simulink model "Decentralized_Control_G18_2017"  (R2017a)
settings: Solver=VariableStepAuto  StartTime=0.0  StopTime=35  RelTol=1e-3
values from neighbouring files (symbols this model uses):
  DH = Robot_G18()    [Kinematics_G18.m]
undefined symbols (not defined in the file or in its folder): DK_dH, DK_pH
libraries: vrlib x7, simulink_extras x3, dspinverses x2, aerolibanimutils x1, RobotG18_Blocos x1, simulink x1
settings Model: Creator=Ricardo Henriques  LastModifiedBy=Catarina
settings OptimizationCC: LifeSpan=inf

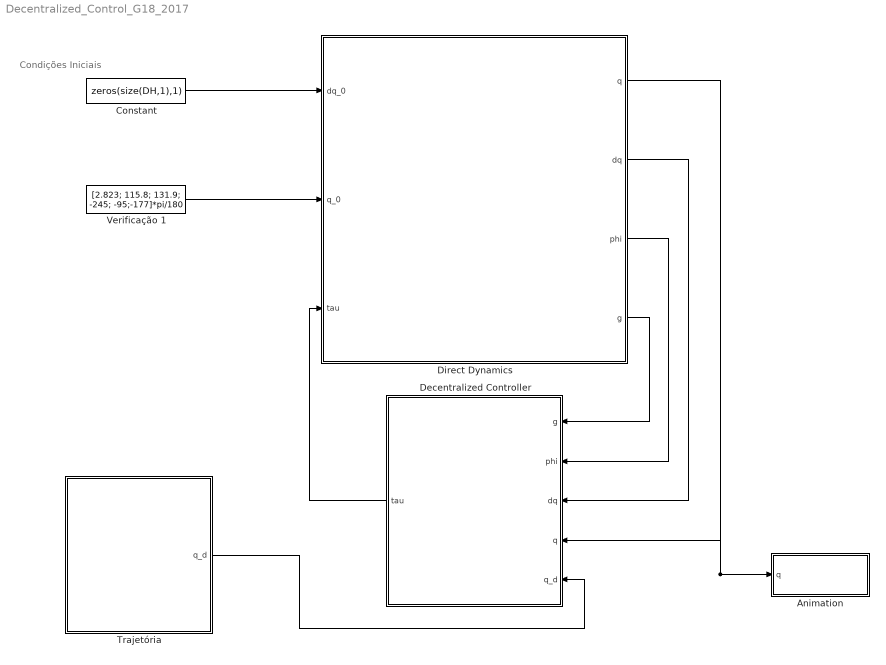
== system Decentralized_Control_G18_2017 ==
  note: Condições Iniciais
  "Animation " : Subsystem
  Constant : Constant  Value=zeros(size(DH,1),1)  VectorParams1D=off
  Decentralized Controller : Subsystem
  Direct Dynamics : Subsystem
  Trajetória : Subsystem
  Verificação 1 : Constant  Value=[2.823; 115.8; 131.9; -245; -95;-177]*pi/180  VectorParams1D=off
  wires:
  Constant/1 -> Direct Dynamics/1(dq_0)
  Direct Dynamics/4(g) -> Decentralized Controller/1(g)
  Direct Dynamics/3(phi) -> Decentralized Controller/2("phi ")
  Decentralized Controller/1(tau) -> Direct Dynamics/3(tau)
  Trajetória/1(q_d) -> Decentralized Controller/5(q_d)
  Verificação 1/1 -> Direct Dynamics/2(q_0)
  Direct Dynamics/2(dq) -> Decentralized Controller/3(dq)
  Direct Dynamics/1(q) -> Decentralized Controller/4(q), "Animation "/1("q ")

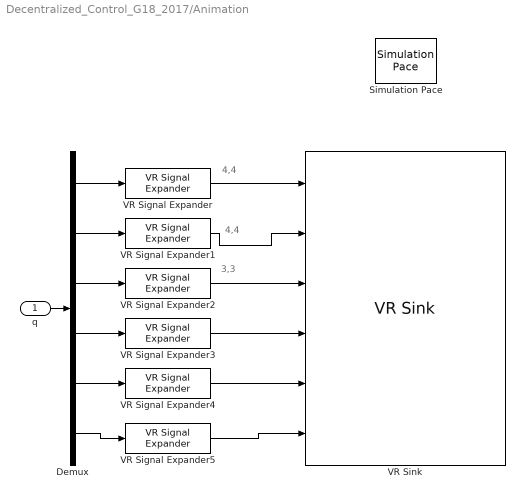
== system Decentralized_Control_G18_2017/Animation  ==
  note: 4,4
  note: 3,3
  note: 4,4
  "q " : Inport
  Demux : Demux  Outputs=6
  Simulation Pace : aerolibanimutils/Simulation Pace  SimulationPace=1  SleepMode=Auto  OutputPaceError=off  SampleTime=1/30
  VR Signal Expander{,1..5} (6 alike) : vrlib/VR Signal Expander  outwidth=4  outidx=4
  VR Sink : vrlib/VR Sink  InstantiateOnLoad=on  SampleTime=1/30  ViewEnable=on  RemoteChange=off  RemoteView=off  FieldsWritten=Jt1_DH_dv.rotation.4.1.1.double#Jt2_DH_dv.rotation.4.1.1.double#Jt3_DH_dv.rotation.4.1.1.double#Jt4_DH_dv.rotation.4.1.1.double#Jt5_DH_dv.rotation.4.1.1.double#Jt6_DH_dv.rotation.4.1.1.double  WorldFileName=RobotG18_Opt_NoAxes.wrl  WorldDescription=D-H Reference Frames for Virtual Reality Robot  AutoView=off  VideoDimensions=[]  AllowVariableSize=off
  wires:
  "q "/1 -> Demux/1
  Demux/1 -> VR Signal Expander/1
  Demux/2 -> VR Signal Expander1/1
  Demux/3 -> VR Signal Expander2/1
  Demux/4 -> VR Signal Expander3/1
  Demux/5 -> VR Signal Expander4/1
  Demux/6 -> VR Signal Expander5/1
  VR Signal Expander/1 -> VR Sink/1
  VR Signal Expander1/1 -> VR Sink/2
  VR Signal Expander5/1 -> VR Sink/6
  VR Signal Expander2/1 -> VR Sink/3
  VR Signal Expander3/1 -> VR Sink/4
  VR Signal Expander4/1 -> VR Sink/5

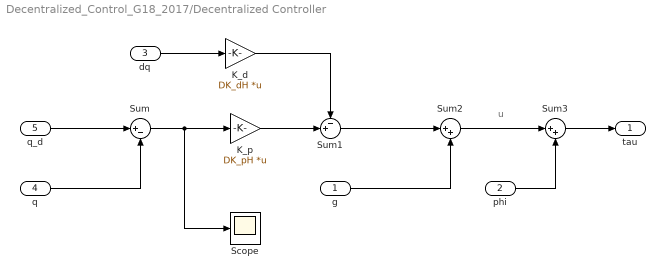
== system Decentralized_Control_G18_2017/Decentralized Controller ==
  note: u
  g : Inport
  "phi " : Inport  Port=2
  dq : Inport  Port=3
  q : Inport  Port=4
  q_d : Inport  Port=5
  K_d : Gain  Gain=DK_dH  Multiplication=Matrix(K*u) (u vector)
  K_p : Gain  Gain=DK_pH  Multiplication=Matrix(K*u) (u vector)
  Scope : Scope
  Sum : Sum  Inputs=|+-
  Sum1 : Sum  Inputs=-+|
  Sum2 : Sum  Inputs=|++
  Sum3 : Sum  Inputs=|++
  tau : Outport
  wires:
  q_d/1 -> Sum/1
  Sum1/1 -> Sum2/1
  g/1 -> Sum2/2
  Sum3/1 -> tau/1
  "phi "/1 -> Sum3/2
  Sum2/1 -> Sum3/1
  q/1 -> Sum/2
  dq/1 -> K_d/1
  K_d/1 -> Sum1/1
  K_p/1 -> Sum1/2
  Sum/1 -> Scope/1, K_p/1

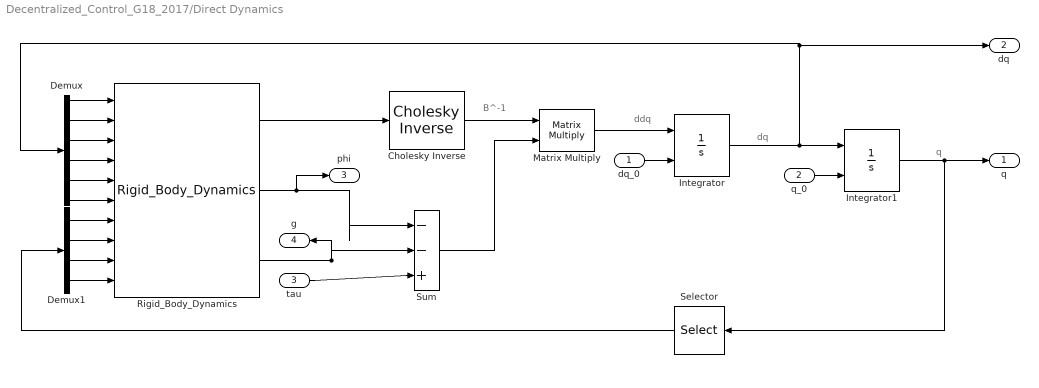
== system Decentralized_Control_G18_2017/Direct Dynamics ==
  note: q
  note: dq
  note: ddq
  note: B^-1
  dq_0 : Inport
  q_0 : Inport  Port=2
  tau : Inport  Port=3
  Cholesky Inverse : dspinverses/Cholesky Inverse  errmode=Warning
      settings: SourceProductBaseCode=DS
  Demux : Demux  Outputs=6
  Demux1 : Demux
  Integrator : Integrator  InitialConditionSource=external
  Integrator1 : Integrator  InitialConditionSource=external
  Matrix Multiply : Product  Multiplication=Matrix(*)
  Rigid_Body_Dynamics : RobotG18_Blocos/Rigid_Body_Dynamics  SystemSampleTime=-1  Latency=0  AutoFrameSizeCalculation=off
  Selector : Selector  InputPortWidth=6  IndexOptions=Index vector (dialog)  Indices=[2 3 4 5]  OutputSizes=1
  Sum : Sum  Inputs=|--+
  q : Outport
  dq : Outport  Port=2
  phi : Outport  Port=3
  g : Outport  Port=4
  wires:
  dq_0/1 -> Integrator/2
  Integrator1/1 -> q/1, Selector/1
  Integrator/1 -> Demux/1, dq/1, Integrator1/1
  q_0/1 -> Integrator1/2
  Matrix Multiply/1 -> Integrator/1
  Cholesky Inverse/1 -> Matrix Multiply/1
  Sum/1 -> Matrix Multiply/2
  Rigid_Body_Dynamics/1 -> Cholesky Inverse/1
  tau/1 -> Sum/3
  Rigid_Body_Dynamics/3 -> g/1, Sum/2
  Rigid_Body_Dynamics/2 -> phi/1, Sum/1
  Demux/1 -> Rigid_Body_Dynamics/1
  Demux/2 -> Rigid_Body_Dynamics/2
  Demux/3 -> Rigid_Body_Dynamics/3
  Demux/4 -> Rigid_Body_Dynamics/4
  Demux/5 -> Rigid_Body_Dynamics/5
  Demux/6 -> Rigid_Body_Dynamics/6
  Demux1/1 -> Rigid_Body_Dynamics/7
  Demux1/2 -> Rigid_Body_Dynamics/8
  Demux1/3 -> Rigid_Body_Dynamics/9
  Demux1/4 -> Rigid_Body_Dynamics/10
  Selector/1 -> Demux1/1

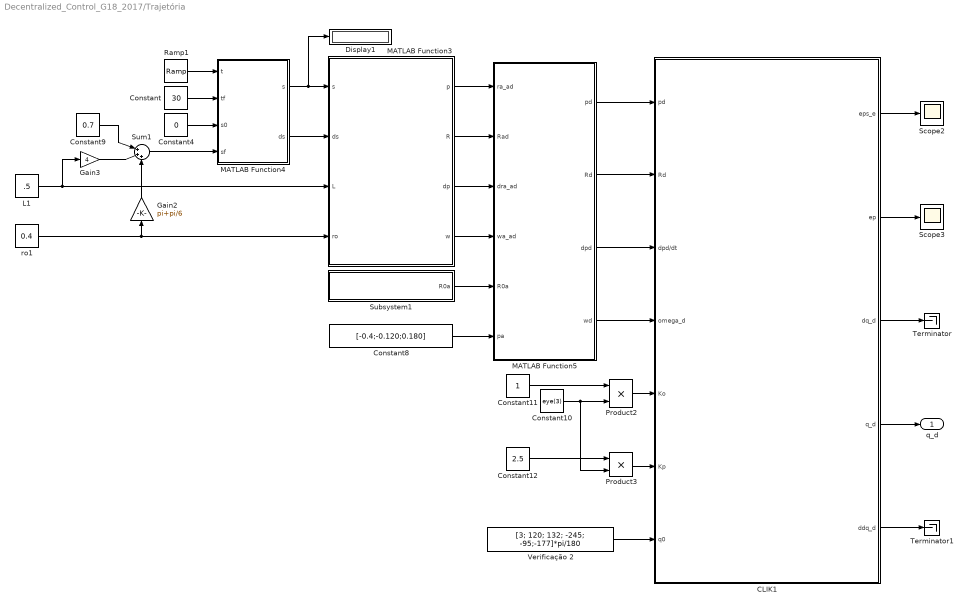
== system Decentralized_Control_G18_2017/Trajetória ==
  CLIK1 : Subsystem
  Constant : Constant  Value=30
  Constant10 : Constant  Value=eye(3)
  Constant11 : Constant
  Constant12 : Constant  Value=2.5
  Constant4 : Constant  Value=0
  Constant8 : Constant  Value=[-0.4;-0.120;0.180]  VectorParams1D=off
  Constant9 : Constant  Value=0.7
  Display1 : Display
  Gain2 : Gain  Gain=pi+pi/6
  Gain3 : Gain  Gain=4
  L1 : Constant  Value=.5
  MATLAB Function3 : MATLAB Function  TreatAsAtomicUnit=on
  MATLAB Function4 : MATLAB Function  TreatAsAtomicUnit=on
  MATLAB Function5 : MATLAB Function  TreatAsAtomicUnit=on
  Product2 : Product
  Product3 : Product
  Ramp1 : simulink/Sources/Ramp  slope=1  start=0  X0=0
  Scope2 : Scope
  Scope3 : Scope
  Subsystem1 : Subsystem
  Sum1 : Sum  Inputs=|+++
  Terminator : Terminator
  Terminator1 : Terminator
  Verificação 2 : Constant  Value=[3; 120; 132; -245; -95;-177]*pi/180  VectorParams1D=off  SampleTime=inf
  ro1 : Constant  Value=0.4
  q_d : Outport
  wires:
  MATLAB Function5/4(wd) -> CLIK1/4(omega_d)
  Constant8/1 -> MATLAB Function5/6(pa)
  Constant10/1 -> Product3/2, Product2/2
  CLIK1/4(q_d) -> q_d/1
  CLIK1/2(ep) -> Scope3/1
  MATLAB Function5/3(dpd) -> CLIK1/3(dpd/dt)
  CLIK1/1(eps_e) -> Scope2/1
  Product2/1 -> CLIK1/5(Ko)
  MATLAB Function3/3(dp) -> MATLAB Function5/3(dra_ad)
  ro1/1 -> MATLAB Function3/4(ro), Gain2/1
  MATLAB Function4/2(ds) -> MATLAB Function3/2(ds)
  Constant9/1 -> Sum1/1
  Constant4/1 -> MATLAB Function4/3(s0)
  Sum1/1 -> MATLAB Function4/4(sf)
  MATLAB Function5/1(pd) -> CLIK1/1(pd)
  L1/1 -> MATLAB Function3/3(L), Gain3/1
  Constant/1 -> MATLAB Function4/2(tf)
  MATLAB Function4/1(s) -> Display1/1, MATLAB Function3/1(s)
  Gain2/1 -> Sum1/3
  MATLAB Function3/4(w) -> MATLAB Function5/4(wa_ad)
  Ramp1/1 -> MATLAB Function4/1(t)
  MATLAB Function5/2(Rd) -> CLIK1/2(Rd)
  Gain3/1 -> Sum1/2
  Constant12/1 -> Product3/1
  MATLAB Function3/1(p) -> MATLAB Function5/1(ra_ad)
  MATLAB Function3/2(R) -> MATLAB Function5/2(Rad)
  Product3/1 -> CLIK1/6(Kp)
  Constant11/1 -> Product2/1
  Subsystem1/1(R0a) -> MATLAB Function5/5(R0a)
  Verificação 2/1 -> CLIK1/7(q0)
  CLIK1/3(dq_d) -> Terminator/1
  CLIK1/5(ddq_d) -> Terminator1/1

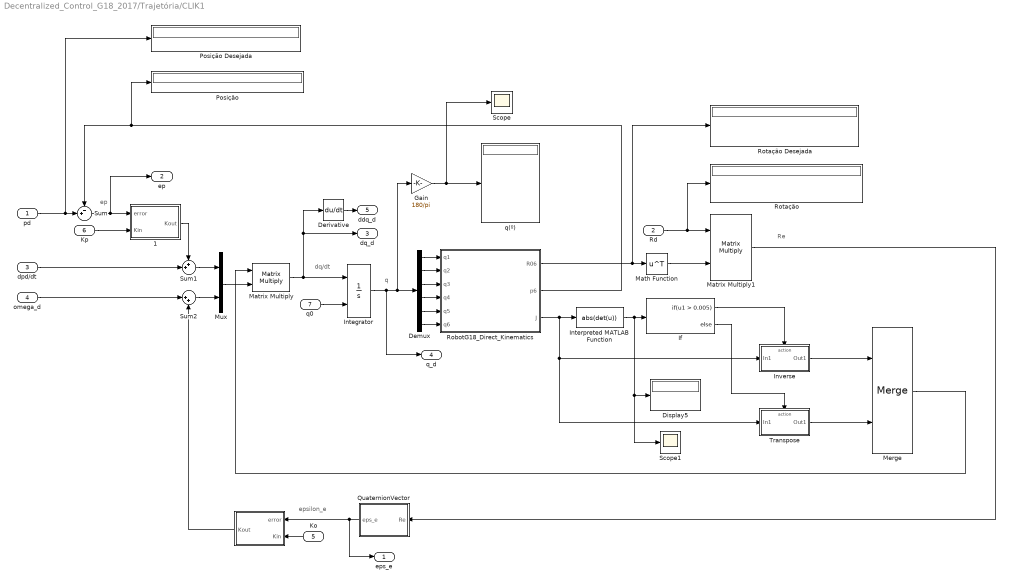
== system Decentralized_Control_G18_2017/Trajetória/CLIK1 ==
  note: epsilon_e
  note: Re
  note: ep
  note: dq/dt
  note: q
  pd : Inport
  Rd : Inport  Port=2
  dpd/dt : Inport  Port=3
  omega_d : Inport  Port=4
  Ko : Inport  Port=5
  Kp : Inport  Port=6
  q0 : Inport  Port=7
  " " : MATLAB Function  TreatAsAtomicUnit=on
  " 1" : MATLAB Function  TreatAsAtomicUnit=on
  Demux : Demux  Outputs=6
  Derivative : Derivative
  Display5 : Display
  Gain : Gain  Gain=180/pi
  If : If  IfExpression=u1 > 0.005  ZeroCross=off
  Integrator : Integrator  InitialConditionSource=external
  Interpreted MATLAB Function : MATLABFcn  MATLABFcn=abs(det(u))
  Inverse : Subsystem  TreatAsAtomicUnit=on
  Math Function : Math  Operator=transpose  SaturateOnIntegerOverflow=on
  Matrix Multiply : Product  Multiplication=Matrix(*)
  Matrix Multiply1 : Product  Multiplication=Matrix(*)
  Merge : Merge
  Mux : Mux  Inputs=2
  Posição : Display
      settings: Decimation=3
  Posição Desejada : Display
      settings: Decimation=3
  QuaternionVector : MATLAB Function  TreatAsAtomicUnit=on
  RobotG18_Direct_Kinematics : MATLAB Function  TreatAsAtomicUnit=on
  Rotação : Display
      settings: Decimation=3
  Rotação Desejada : Display
      settings: Decimation=3
  Scope : Scope
  Scope1 : Scope
  Sum : Sum  Inputs=-+|
  Sum1 : Sum  Inputs=++|
  Sum2 : Sum  Inputs=|++
  Transpose : Subsystem  TreatAsAtomicUnit=on
  q(º) : Display
  eps_e : Outport
  ep : Outport  Port=2
  dq_d : Outport  Port=3
  q_d : Outport  Port=4
  ddq_d : Outport  Port=5
  wires:
  Integrator/1 -> q_d/1, Gain/1, Demux/1
  Demux/3 -> RobotG18_Direct_Kinematics/3(q3)
  Demux/4 -> RobotG18_Direct_Kinematics/4(q4)
  Demux/1 -> RobotG18_Direct_Kinematics/1(q1)
  Demux/2 -> RobotG18_Direct_Kinematics/2(q2)
  Demux/5 -> RobotG18_Direct_Kinematics/5(q5)
  Demux/6 -> RobotG18_Direct_Kinematics/6(q6)
  QuaternionVector/1(eps_e) -> " "/1(error), eps_e/1
  Matrix Multiply/1 -> Derivative/1, dq_d/1, Integrator/1
  Math Function/1 -> Matrix Multiply1/2
  " "/1(Kout) -> Sum2/2
  omega_d/1 -> Sum2/1
  Sum2/1 -> Mux/2
  Sum1/1 -> Mux/1
  Mux/1 -> Matrix Multiply/2
  Rd/1 -> Rotação/1, Matrix Multiply1/1
  Matrix Multiply1/1 -> QuaternionVector/1(Re)
  pd/1 -> Posição Desejada/1, Sum/2
  RobotG18_Direct_Kinematics/2(p6) -> Posição/1, Sum/1
  Sum/1 -> " 1"/1(error), ep/1
  dpd/dt/1 -> Sum1/2
  RobotG18_Direct_Kinematics/1(R06) -> Math Function/1, Rotação Desejada/1
  RobotG18_Direct_Kinematics/3(J) -> Interpreted MATLAB Function/1, Inverse/1(In1), Transpose/1(In1)
  If/1 -> Inverse/Action
  If/2 -> Transpose/Action
  Transpose/1(Out1) -> Merge/2
  Inverse/1(Out1) -> Merge/1
  Merge/1 -> Matrix Multiply/1
  Gain/1 -> Scope/1, q(º)/1
  q0/1 -> Integrator/2
  Ko/1 -> " "/2(Kin)
  " 1"/1(Kout) -> Sum1/1
  Kp/1 -> " 1"/2(Kin)
  Interpreted MATLAB Function/1 -> Scope1/1, Display5/1, If/1
  Derivative/1 -> ddq_d/1

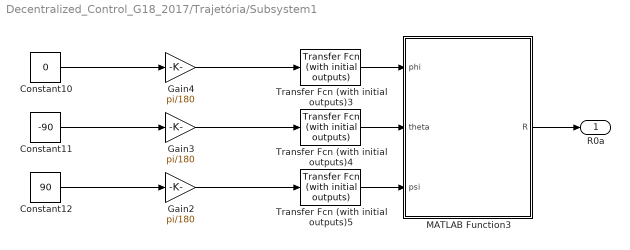
== system Decentralized_Control_G18_2017/Trajetória/Subsystem1 ==
  Constant10 : Constant  Value=0
  Constant11 : Constant  Value=-90
  Constant12 : Constant  Value=90
  Gain2 : Gain  Gain=pi/180
  Gain3 : Gain  Gain=pi/180
  Gain4 : Gain  Gain=pi/180
  MATLAB Function3 : MATLAB Function  TreatAsAtomicUnit=on
  Transfer Fcn (with initial outputs)3 : simulink_extras/Additional Linear/Transfer Fcn (with initial outputs)  N=[2]  D="[1  2]"  Y0=0  U0=0
  Transfer Fcn (with initial outputs)4 : simulink_extras/Additional Linear/Transfer Fcn (with initial outputs)  N=[2]  D="[1  2]"  Y0=-90  U0=0
  Transfer Fcn (with initial outputs)5 : simulink_extras/Additional Linear/Transfer Fcn (with initial outputs)  N=[2]  D="[1  2]"  Y0=90  U0=0
  R0a : Outport
  wires:
  Gain3/1 -> Transfer Fcn (with initial outputs)4/1
  Gain2/1 -> Transfer Fcn (with initial outputs)5/1
  Gain4/1 -> Transfer Fcn (with initial outputs)3/1
  Constant10/1 -> Gain4/1
  Transfer Fcn (with initial outputs)4/1 -> MATLAB Function3/2(theta)
  Transfer Fcn (with initial outputs)5/1 -> MATLAB Function3/3(psi)
  Transfer Fcn (with initial outputs)3/1 -> MATLAB Function3/1(phi)
  Constant11/1 -> Gain3/1
  Constant12/1 -> Gain2/1
  MATLAB Function3/1(R) -> R0a/1

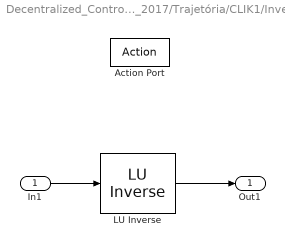
== system Decentralized_Control_G18_2017/Trajetória/CLIK1/Inverse ==
  In1 : Inport
  Action Port : ActionPort
  " LU Inverse" : dspinverses/ LU Inverse
  Out1 : Outport
  wires:
  In1/1 -> " LU Inverse"/1
  " LU Inverse"/1 -> Out1/1

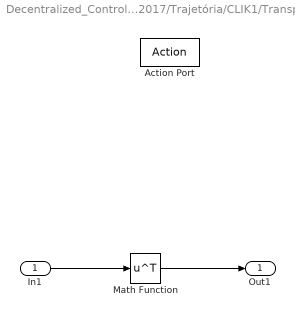
== system Decentralized_Control_G18_2017/Trajetória/CLIK1/Transpose ==
  In1 : Inport
  Action Port : ActionPort
  Math Function : Math  Operator=transpose  SaturateOnIntegerOverflow=on
  Out1 : Outport
  wires:
  In1/1 -> Math Function/1
  Math Function/1 -> Out1/1

== matlab function Decentralized_Control_G18_2017/Trajetória/CLIK1/  ==
  data: error input; Kin input; Kout output
function Kout = Gains(error, Kin)

Kout = Kin*error;

== matlab function Decentralized_Control_G18_2017/Trajetória/CLIK1/ 1 ==
  data: error input; Kin input; Kout output
function Kout = Gains(error, Kin)

Kout = Kin*error;

== matlab function Decentralized_Control_G18_2017/Trajetória/CLIK1/QuaternionVector ==
  data: Re input; eps_e output
function eps_e  = QuaternionVector(Re)

eps_e = 0.5 * [sign(Re(3,2)-Re(2,3)) * sqrt(abs(Re(1,1)-Re(2,2)-Re(3,3)+1));
               sign(Re(1,3)-Re(3,1)) * sqrt(abs(Re(2,2)-Re(1,1)-Re(3,3)+1));
               sign(Re(2,1)-Re(1,2)) * sqrt(abs(Re(3,3)-Re(1,1)-Re(2,2)+1))];
           
end

== matlab function Decentralized_Control_G18_2017/Trajetória/CLIK1/RobotG18_Direct_Kinematics ==
  data: q1 input; R06 output; q2 input; q3 input; q4 input; q5 input; q6 input; p6 output; J output
function [R06,p6,J] = RobotG18_Direct_Kinematics(q1,q2,q3,q4,q5,q6)
%#codegen

%    This function was generated by the Symbolic Math Toolbox version 7.0.
%    15-Apr-2021 18:49:51

t2 = q2+q3+q4;
t3 = cos(q1);
t4 = sin(q6);
t5 = sin(q1);
t6 = sin(q5);
t7 = t5.*t6;
t8 = cos(t2);
t9 = cos(q5);
t10 = t7-t3.*t8.*t9;
t11 = sin(t2);
t12 = cos(q6);
t13 = t3.*t6;
t14 = t5.*t8.*t9;
t15 = t13+t14;
t16 = q2+q3;
t17 = cos(q2);
t18 = sin(q2);
t19 = sin(q3);
t20 = cos(t16);
t21 = sin(q4);
t22 = sin(t16);
t23 = cos(q4);
t24 = cos(q3);
t25 = t5.*t17.*(1.7e1./4.0e1);
t26 = t5.*t6.*t8.*(4.1e1./5.0e2);
t27 = t5.*t17.*t24.*(4.9e1./1.25e2);
t28 = t22.*(4.9e1./1.25e2);
t29 = t18.*(1.7e1./4.0e1);
t30 = t20.*t21.*(4.1e1./5.0e2);
t31 = t22.*t23.*(4.1e1./5.0e2);
t32 = t30+t31;
t33 = t6.*t32;
t34 = t20.*t23.*(1.9e1./2.0e2);
t35 = t8.*(1.9e1./2.0e2);
t36 = t6.*t11.*(4.1e1./5.0e2);
t37 = t5.*(1.09e2./1.0e3);
t38 = t3.*t17.*(1.7e1./4.0e1);
t39 = t5.*t9.*(4.1e1./5.0e2);
t40 = t3.*t6.*t8.*(4.1e1./5.0e2);
t41 = t3.*t17.*t24.*(4.9e1./1.25e2);
t42 = t37+t38+t39+t40+t41-t3.*t18.*t19.*(4.9e1./1.25e2)-t3.*t20.*t21.*(1.9e1./2.0e2)-t3.*t22.*t23.*(1.9e1./2.0e2);
t43 = t28+t29+t33+t34-t21.*t22.*(1.9e1./2.0e2);
t44 = t28+t35+t36;
t45 = t35+t36;
t46 = q2+q3+q4+q5;
t47 = sin(t46);
t48 = t47.*(4.1e1./1.0e3);
t49 = t20.*(4.9e1./1.25e2);
t50 = q2+q3+q4-q5;
t51 = sin(t50);
t52 = t5.*t9;
t53 = t3.*t6.*t8;
t54 = t52+t53;
t55 = t5.*t6.*t8;
t56 = t55-t3.*t9;
t57 = t6.*t11;
R06 = reshape([-t10.*t12-t3.*t4.*t11,t12.*t15-t4.*t5.*t11,t4.*t8+t9.*t11.*t12,t4.*t10-t3.*t11.*t12,-t4.*t15-t5.*t11.*t12,t8.*t12-t4.*t9.*t11,t54,t56,t57],[3,3]);
if nargout > 1
    p6 = [t42;t3.*(-1.09e2./1.0e3)+t25+t26+t27-t3.*t9.*(4.1e1./5.0e2)-t5.*t18.*t19.*(4.9e1./1.25e2)-t5.*t20.*t21.*(1.9e1./2.0e2)-t5.*t22.*t23.*(1.9e1./2.0e2);t28+t29+t33+t34-t21.*t22.*(1.9e1./2.0e2)+8.9e1./1.0e3];
end
if nargout > 2
    J = reshape([t3.*(1.09e2./1.0e3)-t25-t26-t27+t3.*t9.*(4.1e1./5.0e2)+t5.*t18.*t19.*(4.9e1./1.25e2)+t5.*t20.*t21.*(1.9e1./2.0e2)+t5.*t22.*t23.*(1.9e1./2.0e2),t42,0.0,0.0,0.0,1.0,-t3.*t43,-t5.*t43,t11.*(-1.9e1./2.0e2)+t17.*(1.7e1./4.0e1)+t48+t49-t51.*(4.1e1./1.0e3),t5,-t3,0.0,-t3.*t44,-t5.*t44,t11.*(-1.9e1./2.0e2)+t48+t49-t51.*(4.1e1./1.0e3),t5,-t3,0.0,-t3.*t45,-t5.*t45,t11.*(-1.9e1./2.0e2)+t48-t51.*(4.1e1./1.0e3),t5,-t3,0.0,t5.*t6.*(-4.1e1./5.0e2)-t3.*t9.*t17.*t19.*t21.*(4.1e1./5.0e2)-t3.*t9.*t18.*t19.*t23.*(4.1e1./5.0e2)-t3.*t9.*t18.*t21.*t24.*(4.1e1./5.0e2)+t3.*t9.*t17.*t23.*t24.*(4.1e1./5.0e2),t3.*t6.*(4.1e1./5.0e2)-t5.*t9.*t17.*t19.*t21.*(4.1e1./5.0e2)-t5.*t9.*t18.*t19.*t23.*(4.1e1./5.0e2)-t5.*t9.*t18.*t21.*t24.*(4.1e1./5.0e2)+t5.*t9.*t17.*t23.*t24.*(4.1e1./5.0e2),t48+t51.*(4.1e1./1.0e3),-t3.*t11,-t5.*t11,t8,0.0,0.0,0.0,t54,t56,t57],[6,6]);
end

== matlab function Decentralized_Control_G18_2017/Trajetória/MATLAB Function3 ==
  data: p output; R output; s input; ds input; L input; ro input; dp output; w output
function [p,R,dp,w] = trajectory(s,ds,L,ro)

p=zeros(3,1);
R=eye(3);
dp=zeros(3,1);
w=zeros(3,1);

if 0 <= s && s<= L
%% Path 1 ------- Subida ---------
    p=[0;-s;0];
    R=[1 0 0; 0 1 0; 0 0 1];
    
    dp=[0;ds;0];
    w=zeros(3,1);
    
elseif L < s && s <= L+((pi/2)*ro)
%% Path 2  ------- Roda ---------
    p=[ro*sin((s-L)/ro);
        -L;
        -ro+ro*cos((s-L)/ro)];
    
    R=[ cos((s-L)/ro)   0   sin((s-L)/ro);
        0          1          0
        -sin((s-L)/ro)   0    cos((s-L)/ro)];
    
    dp = ds*[cos((s-L)/ro);0;-sin((s-L)/ro)];
    
    dR = (ds/ro)*[-sin((s-L)/ro)  0  -cos((s-L)/ro);
        0          1       0
        cos((s-L)/ro)   0  -sin((s-L)/ro)];
    Sw=dR*R';
    
    w = [Sw(3,2);Sw(1,3);Sw(2,1)];
    
elseif L+((pi/2)*ro) < s && s <= (2*L+((pi/2)*ro))
%% Path 3  ------- Descida ---------
    p = [ro;s-((2*L)+((pi/2)*ro));-ro];
    R = [0 0 1; 0 1 0; -1 0 0];
    
    dp = [ro;ds;-ro];
    w = zeros(3,1);
    
elseif (2*L+((pi/2)*ro)) < s && s <= (2*L+((pi/2)*ro))+0.2
%% Path 4   ------- Estica (Coloca produto) ---------
    p = [(s-((2*L)+((pi/2)*ro)))+ro;0;-ro];
    R = [0 0 1; 0 1 0; -1 0 0];
    
    dp = [ro;ds;-ro];
    w = zeros(3,1);
    
elseif (2*L+((pi/2)*ro))+0.2 < s && s <= (2*L+((pi/2)*ro))+0.5
%% Path 4  ------- Tempo de espera (larga produto) ---------
    p = [ro+0.2;0;-ro];
    R = [0 0 1; 0 1 0; -1 0 0];
    
    dp = [ro;ds;-ro];
    w = zeros(3,1);
    
elseif (2*L+((pi/2)*ro))+0.5 < s && s <= (2*L+((pi/2)*ro)+0.7)
%% Path 5   ------- Recolhe ---------
    p = [-(s-((2*L)+((pi/2)*ro)+0.7))+ro;0;-ro];
    R = [0 0 1; 0 1 0; -1 0 0];
    
    dp = [ro;ds;-ro];
    w = zeros(3,1);
    
elseif (2*L+((pi/2)*ro)+0.7) < s && s <= (3*L+((pi/2)*ro)+0.7)
    %% Path 4   ------- Subida ---------
    p = [ro;-(s-(2*L+((pi/2)*ro)+0.7));-ro];
    R = [0 0 1; 0 1 0; -1 0 0];
    
    dp = [ro;ds;-ro];
    w = zeros(3,1);
    

elseif (3*L+((pi/2)*ro)+0.7) < s && s <= (3*L+2*((pi/2+pi/12)*ro)+0.7)
%% Path 5      ------- Roda de volta ---------
    p=[ro*sin(-(s-L-0.7)/ro);
        -L;
        -ro+ro*cos(-(s-L-0.7)/ro)];
    
    R=[ cos((s-L-0.7)/ro)   0   -sin((s-L-0.7)/ro);
        0          1          0
        sin((s-L-0.7)/ro)   0    cos((s-L-0.7)/ro)];
    
    dp = ds*[cos((s-L-0.7)/ro);0;-sin((s-L-0.7)/ro)];
    
    dR = (ds/ro)*[-sin((s-L-0.7)/ro)  0  -cos((s-L-0.7)/ro);
        0          1       0
        cos((s-L-0.7)/ro)   0  -sin((s-L-0.7)/ro)];
    Sw=dR*R';
    
    w = [Sw(3,2);Sw(1,3);Sw(2,1)];
    

elseif (3*L+2*((pi/2+pi/12)*ro)+0.7) < s && s <= (4*L+2*((pi/2+pi/12)*ro)+0.7)
%% Path 6  ------- Descida ---------
    p=[0;s-(4*L+2*((pi/2+pi/12)*ro)+0.7);0];
    R=[1 0 0; 0 1 0; 0 0 1];
    
    dp=[0;ds;0];
    w=zeros(3,1);
    
end
end

== matlab function Decentralized_Control_G18_2017/Trajetória/MATLAB Function4 ==
  data: t input; s output; tf input; s0 input; sf input; ds output
function [s,ds] = length(t,tf,s0,sf)
if t<=tf
    s=s0+3*(sf-s0)*(t/tf)^2-2*(sf-s0)*(t/tf)^3;
    
    ds = 6*(sf-s0)*t/tf^2-6*(sf-s0)*t^2/tf^3;
else
    s=sf;
    ds=0;
end
end

== matlab function Decentralized_Control_G18_2017/Trajetória/MATLAB Function5 ==
  data: ra_ad input; pd output; Rad input; dra_ad input; wa_ad input; R0a input; pa input; Rd output; dpd output; wd output
function [pd,Rd,dpd,wd]=fcn(ra_ad,Rad,dra_ad,wa_ad,R0a,pa)

pd = pa+R0a*ra_ad;
Rd = R0a*Rad;
dpd = R0a*dra_ad;
wd = R0a*wa_ad;

== matlab function Decentralized_Control_G18_2017/Trajetória/Subsystem1/MATLAB Function3 ==
  data: phi input; R output; theta input; psi input
function R  = matriz_R(phi, theta,psi)

s_x = sin(phi);
s_y = sin(theta);
s_z = sin(psi);

c_x = cos(phi);
c_y = cos(theta);
c_z = cos(psi);
 
R = [(c_x*c_y*c_z)-(s_x*s_z)    -(c_x*c_y*s_z)-(s_x*c_z)  c_x*s_y;
     (s_x*c_y*c_z)+(c_x*s_z)    -(s_x*c_y*s_z)+(c_x*c_z)  s_x*s_y;
     -s_y*c_z                    s_y*s_z                  c_y    ];
end
